simulink model "Stirred_tank_heater_FLC_Xilinx"  (R2017b)
settings: Solver=VariableStepAuto  StartTime=0.0  StopTime=4  RelTol=1e-3
libraries: xbsIndex_r4 x251
(part 1 of 2)
settings Model: Creator=HP  LastModifiedBy=HP

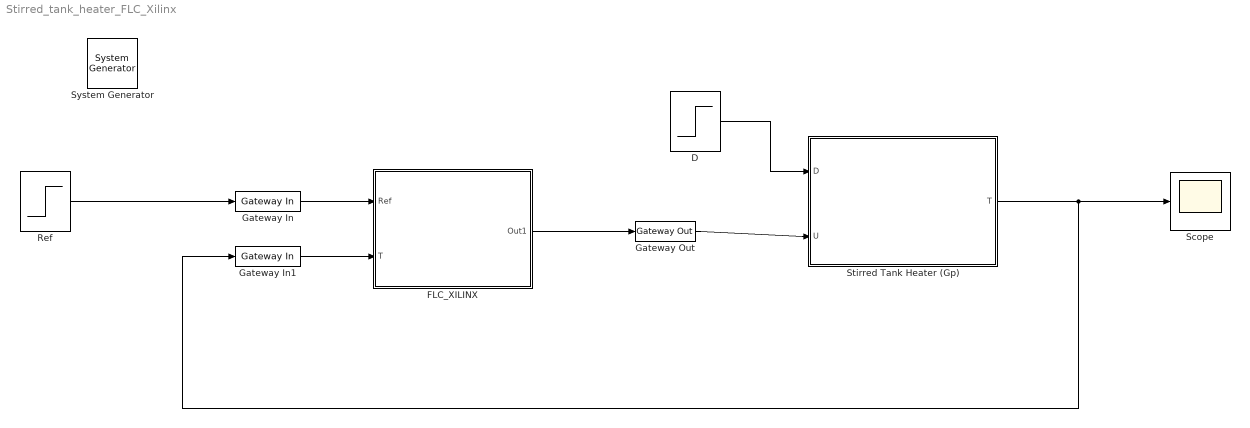
== system Stirred_tank_heater_FLC_Xilinx ==
  " System Generator" : xbsIndex_r4/ System Generator  Tag=genX  xilinxfamily=kintex7  part=xc7k325t  speed=-3  package=fbg676  synthesis_tool=Vivado  clock_wrapper=Clock Enables  directory=./netlist  proj_type=Vivado  Synth_file=Vivado Synthesis Defaults  Impl_file=Vivado Implementation Defaults  testbench=off  simulink_period=1/10e4  sysclk_period=10  dcm_input_clock_period=10  incr_netlist=off  trim_vbits=Everywhere in SubSystem  dbl_ovrd=According to Block Masks  core_generation=According to Block Masks  run_coregen=off  deprecated_control=off  eval_field=0  block_type=sysgen
  D : Step  Time=2  After=0  SampleTime=0.01
  FLC_XILINX : Subsystem
  Gateway In : xbsIndex_r4/Gateway In  gui_display_data_type=Floating-point  arith_type=Floating-point  n_bits=16  bin_pt=14  preci_type=Double  exp_width=8  frac_width=24  rows=1  columns=1  quantization="Round  (unbiased: +/- Inf)"  overflow=Saturate  period=1/10e4  UseAsADC=off  ADCChannel='1'  interface=None  automatic_assignment=on  address_offset=hex2dec('00')  intf_name=''  intf_description=''  default_value=0  timing_constraint=None  locs_specified=off  LOCs={}  io_standard={}  inherit_from_input=off  hdl_port=on  dbl_ovrd=off  block_type=gatewayin
  Gateway In1 : xbsIndex_r4/Gateway In  gui_display_data_type=Floating-point  arith_type=Floating-point  n_bits=16  bin_pt=14  preci_type=Double  exp_width=8  frac_width=24  rows=1  columns=1  quantization="Round  (unbiased: +/- Inf)"  overflow=Saturate  period=1/10e4  UseAsADC=off  ADCChannel='1'  interface=None  automatic_assignment=on  address_offset=hex2dec('00')  intf_name=''  intf_description=''  default_value=0  timing_constraint=None  locs_specified=off  LOCs={}  io_standard={}  inherit_from_input=off  hdl_port=on  dbl_ovrd=off  block_type=gatewayin
  Gateway Out : xbsIndex_r4/Gateway Out  inherit_from_input=off  hdl_port=on  rows=1  columns=1  UseAsDAC=off  DACChannel='1'  interface=None  automatic_assignment=on  address_offset=hex2dec('00')  intf_name=''  intf_description=''  timing_constraint=None  locs_specified=off  LOCs={}  io_standard={}  block_type=gatewayout
  Ref : Step  Time=0  SampleTime=0.01
  Scope : Scope
  Stirred Tank Heater (Gp) : Subsystem
  wires:
  FLC_XILINX/1(Out1) -> Gateway Out/1
  Ref/1 -> Gateway In/1
  Gateway In/1 -> FLC_XILINX/1(Ref)
  Stirred Tank Heater (Gp)/1(T) -> Gateway In1/1, Scope/1
  D/1 -> Stirred Tank Heater (Gp)/1(D)
  Gateway Out/1 -> Stirred Tank Heater (Gp)/2(U)
  Gateway In1/1 -> FLC_XILINX/2(T)

== system Stirred_tank_heater_FLC_Xilinx/FLC_XILINX ==
  Ref : Inport
  T : Inport  Port=2
  AddSub2 : xbsIndex_r4/AddSub  mode=Subtraction  use_carryin=off  use_carryout=off  en=off  latency=1  precision=Full  arith_type=Unsigned  n_bits=16  bin_pt=14  quantization=Truncate  overflow=Wrap  use_behavioral_HDL=off  hw_selection=Fabric  pipelined=off  dbl_ovrd=off  block_type=addsub
  CMult1 : xbsIndex_r4/CMult  const=1/12  gui_display_data_type=Floating-point  const_n_bits=16  const_bin_pt=14  float_type=Double  exp_bits=8  fraction_bits=24  en=off  latency=1  precision=Full  arith_type="Signed  (2's comp)"  n_bits=16  bin_pt=14  quantization=Truncate  overflow=Wrap  use_behavioral_HDL=off  mem_type=Distributed RAM  pipeline=off  dbl_ovrd=off  block_type=cmult
  CMult2 : xbsIndex_r4/CMult  const=36  gui_display_data_type=Floating-point  const_n_bits=16  const_bin_pt=14  float_type=Double  exp_bits=8  fraction_bits=24  en=off  latency=1  precision=Full  arith_type="Signed  (2's comp)"  n_bits=16  bin_pt=14  quantization=Truncate  overflow=Wrap  use_behavioral_HDL=off  mem_type=Distributed RAM  pipeline=off  dbl_ovrd=off  block_type=cmult
  CMult3 : xbsIndex_r4/CMult  const=1  gui_display_data_type=Floating-point  const_n_bits=16  const_bin_pt=14  float_type=Double  exp_bits=8  fraction_bits=24  en=off  latency=1  precision=Full  arith_type="Signed  (2's comp)"  n_bits=16  bin_pt=14  quantization=Truncate  overflow=Wrap  use_behavioral_HDL=off  mem_type=Distributed RAM  pipeline=off  dbl_ovrd=off  block_type=cmult
  Deffuzification : Subsystem
  Input Membership func : Subsystem
  Integrator : Subsystem
  Rules decision logic : Subsystem
  derivative : Subsystem
  Out1 : Outport
  wires:
  Input Membership func/4(PS1) -> Rules decision logic/4(PS1)
  Input Membership func/5(PB1) -> Rules decision logic/5(PB1)
  Input Membership func/6(NB2) -> Rules decision logic/6(NB2)
  Input Membership func/8(ZE2) -> Rules decision logic/8(ZE2)
  Rules decision logic/2(NS3) -> Deffuzification/2(NS3)
  Input Membership func/7(NS2) -> Rules decision logic/7(NS2)
  Input Membership func/1(NB1) -> Rules decision logic/1(NB1)
  Rules decision logic/4(PS3) -> Deffuzification/4(PS3)
  Input Membership func/3(ZE1) -> Rules decision logic/3(ZE1)
  Rules decision logic/3(ZE3) -> Deffuzification/3(ZE3)
  Rules decision logic/5(PB3) -> Deffuzification/5(PB3)
  Input Membership func/2(NS1) -> Rules decision logic/2(NS1)
  Input Membership func/10(PB2) -> Rules decision logic/10(PB2)
  Rules decision logic/1(NB3) -> Deffuzification/1(NB3)
  Input Membership func/9(PS2) -> Rules decision logic/9(PS2)
  Deffuzification/1(du) -> CMult2/1
  Integrator/1(u) -> Out1/1
  CMult2/1 -> Integrator/1(du)
  Ref/1 -> AddSub2/1
  AddSub2/1 -> CMult3/1, derivative/1(du)
  T/1 -> AddSub2/2
  CMult1/1 -> Input Membership func/2(de)
  derivative/1(u) -> CMult1/1
  CMult3/1 -> Input Membership func/1(e)

== system Stirred_tank_heater_FLC_Xilinx/Stirred Tank Heater (Gp) ==
  D : Inport
  U : Inport  Port=2
  Add : Sum
  Transfer Fcn : TransferFcn  Numerator=[3]  Denominator=[1 5]
  Transfer Fcn1 : TransferFcn  Numerator=[2]  Denominator=[1 5]
  T : Outport
  wires:
  U/1 -> Transfer Fcn/1
  Add/1 -> T/1
  Transfer Fcn/1 -> Add/2
  Transfer Fcn1/1 -> Add/1
  D/1 -> Transfer Fcn1/1

== system Stirred_tank_heater_FLC_Xilinx/FLC_XILINX/Deffuzification ==
  NB3 : Inport
  NS3 : Inport  Port=2
  ZE3 : Inport  Port=3
  PS3 : Inport  Port=4
  PB3 : Inport  Port=5
  Constant : xbsIndex_r4/Constant  const=0  gui_display_data_type=Floating-point  arith_type=Floating-point  n_bits=16  bin_pt=14  preci_type=Double  exp_width=8  frac_width=24  explicit_period=off  period=1  equ=P=C  opselect=C  inp2=PCIN>>17  opr=+  inp1=P  carry=CIN  dbl_ovrd=off  block_type=constant
  Constant1 : xbsIndex_r4/Constant  const=0  gui_display_data_type=Floating-point  arith_type=Floating-point  n_bits=16  bin_pt=14  preci_type=Double  exp_width=8  frac_width=24  explicit_period=off  period=1  equ=P=C  opselect=C  inp2=PCIN>>17  opr=+  inp1=P  carry=CIN  dbl_ovrd=off  block_type=constant
  Denum : Subsystem
  Denum1 : Subsystem
  Divide : xbsIndex_r4/Divide  flow_control=NonBlocking  axi_optimize_goal=Resources  algorithm_type=Radix2  infoedit1=Specify output fraction-width for Fixed-point division.  fractional_width=16  infoedit2=Specify latency for Floating-point division.  latency=1  rate=1  has_a_tlast=off  has_a_tuser=off  has_b_tlast=off  has_b_tuser=off  en=off  has_result_tready=off  result_tlast_behv=Pass_A_TLAST  has_underflow=off  has_overflow=off  has_invalid_op=off  has_divide_by_zero=off  fpo_op_type=mergeddivide  block_type=divide
      settings: infoedit=Blocking: Wait for data on all inputs, allow back-pressure.<br>NonBlocking: operate every cycle in which all inputs are valid, no back-pressure.
  Mux : xbsIndex_r4/Mux  inputs=2  en=off  latency=1  precision=Full  arith_type=Unsigned  n_bits=16  bin_pt=14  quantization=Truncate  overflow=Wrap  dbl_ovrd=off  block_type=mux
  Relational : xbsIndex_r4/Relational  mode=a!=b  op_type=Bool  en=off  latency=1  dbl_ovrd=off  block_type=relational
  du : Outport
  wires:
  NB3/1 -> Denum/1(NB3), Denum1/1(NB3)
  NS3/1 -> Denum/2(NS3), Denum1/2(NS3)
  PB3/1 -> Denum/5(PB3), Denum1/4(PB3)
  Constant/1 -> Relational/2
  Relational/1 -> Mux/1
  Constant1/1 -> Mux/2
  ZE3/1 -> Denum/3(ZE3)
  PS3/1 -> Denum/4(PS3), Denum1/3(PS3)
  Denum/1(A6) -> Relational/1, Divide/2
  Denum1/1(N) -> Divide/1
  Divide/1 -> Mux/3
  Mux/1 -> du/1

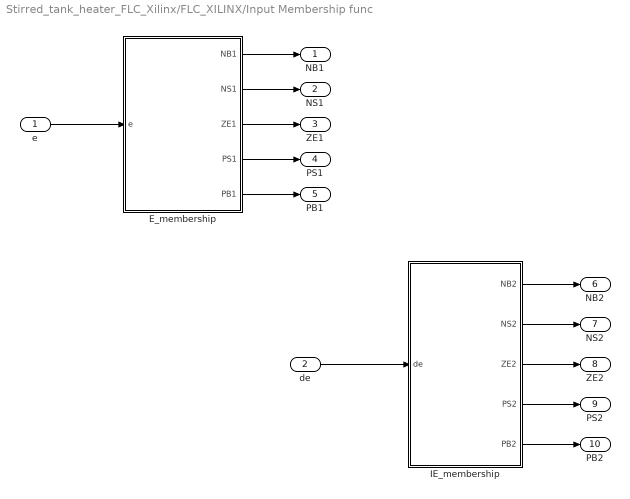
== system Stirred_tank_heater_FLC_Xilinx/FLC_XILINX/Input Membership func ==
  e : Inport
  de : Inport  Port=2
  E_membership : Subsystem
  IE_membership : Subsystem
  NB1 : Outport
  NS1 : Outport  Port=2
  ZE1 : Outport  Port=3
  PS1 : Outport  Port=4
  PB1 : Outport  Port=5
  NB2 : Outport  Port=6
  NS2 : Outport  Port=7
  ZE2 : Outport  Port=8
  PS2 : Outport  Port=9
  PB2 : Outport  Port=10
  wires:
  E_membership/4(PS1) -> PS1/1
  E_membership/2(NS1) -> NS1/1
  E_membership/1(NB1) -> NB1/1
  E_membership/3(ZE1) -> ZE1/1
  e/1 -> E_membership/1(e)
  IE_membership/5(PB2) -> PB2/1
  IE_membership/3(ZE2) -> ZE2/1
  IE_membership/4(PS2) -> PS2/1
  IE_membership/2(NS2) -> NS2/1
  IE_membership/1(NB2) -> NB2/1
  de/1 -> IE_membership/1(de)
  E_membership/5(PB1) -> PB1/1

== system Stirred_tank_heater_FLC_Xilinx/FLC_XILINX/Integrator ==
  du : Inport
  AddSub : xbsIndex_r4/AddSub  mode=Addition  use_carryin=off  use_carryout=off  en=off  latency=0  precision=Full  arith_type=Unsigned  n_bits=16  bin_pt=14  quantization=Truncate  overflow=Wrap  use_behavioral_HDL=off  hw_selection=Fabric  pipelined=off  dbl_ovrd=off  block_type=addsub
  AddSub1 : xbsIndex_r4/AddSub  mode=Addition  use_carryin=off  use_carryout=off  en=off  latency=0  precision=Full  arith_type=Unsigned  n_bits=16  bin_pt=14  quantization=Truncate  overflow=Wrap  use_behavioral_HDL=off  hw_selection=Fabric  pipelined=off  dbl_ovrd=off  block_type=addsub
  CMult : xbsIndex_r4/CMult  const=1/(2*10e4)  gui_display_data_type=Floating-point  const_n_bits=32  const_bin_pt=28  float_type=Double  exp_bits=8  fraction_bits=24  en=off  latency=1  precision=Full  arith_type="Signed  (2's comp)"  n_bits=16  bin_pt=14  quantization=Truncate  overflow=Wrap  use_behavioral_HDL=off  mem_type=Distributed RAM  pipeline=off  dbl_ovrd=off  block_type=cmult
  Delay : xbsIndex_r4/Delay  rst=off  infoeditControl=Selection of Reset will increase slice count due to use of real FFs and instead of SRLs  en=off  latency=1  reg_retiming=off  dbl_ovrd=off  block_type=delay
  Delay1 : xbsIndex_r4/Delay  rst=off  infoeditControl=Selection of Reset will increase slice count due to use of real FFs and instead of SRLs  en=off  latency=1  reg_retiming=off  dbl_ovrd=off  block_type=delay
  u : Outport
  wires:
  CMult/1 -> AddSub1/1
  AddSub1/1 -> u/1, Delay1/1
  AddSub/1 -> CMult/1
  du/1 -> AddSub/1, Delay/1
  Delay/1 -> AddSub/2
  Delay1/1 -> AddSub1/2

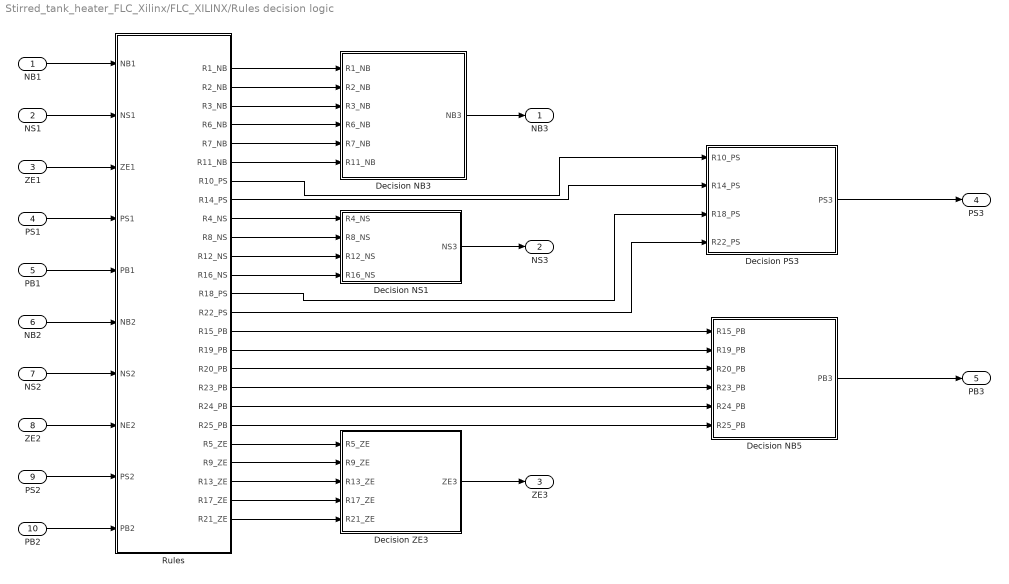
== system Stirred_tank_heater_FLC_Xilinx/FLC_XILINX/Rules decision logic ==
  NB1 : Inport
  NS1 : Inport  Port=2
  ZE1 : Inport  Port=3
  PS1 : Inport  Port=4
  PB1 : Inport  Port=5
  NB2 : Inport  Port=6
  NS2 : Inport  Port=7
  ZE2 : Inport  Port=8
  PS2 : Inport  Port=9
  PB2 : Inport  Port=10
  Decision NB3 : Subsystem
  Decision NB5 : Subsystem
  Decision NS1 : Subsystem
  Decision PS3 : Subsystem
  Decision ZE3 : Subsystem
  Rules : Subsystem
  NB3 : Outport
  NS3 : Outport  Port=2
  ZE3 : Outport  Port=3
  PS3 : Outport  Port=4
  PB3 : Outport  Port=5
  wires:
  NB1/1 -> Rules/1(NB1)
  NB2/1 -> Rules/6(NB2)
  NS2/1 -> Rules/7(NS2)
  ZE2/1 -> Rules/8(NE2)
  PS2/1 -> Rules/9(PS2)
  PB2/1 -> Rules/10(PB2)
  NS1/1 -> Rules/2(NS1)
  ZE1/1 -> Rules/3(ZE1)
  PS1/1 -> Rules/4(PS1)
  PB1/1 -> Rules/5(PB1)
  Decision NB3/1(NB3) -> NB3/1
  Decision NS1/1(NS3) -> NS3/1
  Decision ZE3/1(ZE3) -> ZE3/1
  Decision PS3/1(PS3) -> PS3/1
  Decision NB5/1(PB3) -> PB3/1
  Rules/1(R1_NB) -> Decision NB3/1(R1_NB)
  Rules/2(R2_NB) -> Decision NB3/2(R2_NB)
  Rules/3(R3_NB) -> Decision NB3/3(R3_NB)
  Rules/4(R6_NB) -> Decision NB3/4(R6_NB)
  Rules/5(R7_NB) -> Decision NB3/5(R7_NB)
  Rules/6(R11_NB) -> Decision NB3/6(R11_NB)
  Rules/25(R21_ZE) -> Decision ZE3/5(R21_ZE)
  Rules/24(R17_ZE) -> Decision ZE3/4(R17_ZE)
  Rules/23(R13_ZE) -> Decision ZE3/3(R13_ZE)
  Rules/22(R9_ZE) -> Decision ZE3/2(R9_ZE)
  Rules/21(R5_ZE) -> Decision ZE3/1(R5_ZE)
  Rules/12(R16_NS) -> Decision NS1/4(R16_NS)
  Rules/11(R12_NS) -> Decision NS1/3(R12_NS)
  Rules/10(R8_NS) -> Decision NS1/2(R8_NS)
  Rules/9(R4_NS) -> Decision NS1/1(R4_NS)
  Rules/20(R25_PB) -> Decision NB5/6(R25_PB)
  Rules/19(R24_PB) -> Decision NB5/5(R24_PB)
  Rules/18(R23_PB) -> Decision NB5/4(R23_PB)
  Rules/17(R20_PB) -> Decision NB5/3(R20_PB)
  Rules/16(R19_PB) -> Decision NB5/2(R19_PB)
  Rules/15(R15_PB) -> Decision NB5/1(R15_PB)
  Rules/8(R14_PS) -> Decision PS3/2(R14_PS)
  Rules/7(R10_PS) -> Decision PS3/1(R10_PS)
  Rules/14(R22_PS) -> Decision PS3/4(R22_PS)
  Rules/13(R18_PS) -> Decision PS3/3(R18_PS)

== system Stirred_tank_heater_FLC_Xilinx/FLC_XILINX/derivative ==
  du : Inport
  AddSub2 : xbsIndex_r4/AddSub  mode=Subtraction  use_carryin=off  use_carryout=off  en=off  latency=1  precision=Full  arith_type=Unsigned  n_bits=16  bin_pt=14  quantization=Truncate  overflow=Wrap  use_behavioral_HDL=off  hw_selection=Fabric  pipelined=off  dbl_ovrd=off  block_type=addsub
  CMult2 : xbsIndex_r4/CMult  const=10e4  gui_display_data_type=Floating-point  const_n_bits=16  const_bin_pt=14  float_type=Double  exp_bits=8  fraction_bits=24  en=off  latency=1  precision=Full  arith_type="Signed  (2's comp)"  n_bits=16  bin_pt=14  quantization=Truncate  overflow=Wrap  use_behavioral_HDL=off  mem_type=Distributed RAM  pipeline=off  dbl_ovrd=off  block_type=cmult
  Delay1 : xbsIndex_r4/Delay  rst=off  infoeditControl=Selection of Reset will increase slice count due to use of real FFs and instead of SRLs  en=off  latency=1  reg_retiming=off  dbl_ovrd=off  block_type=delay
  u : Outport
  wires:
  AddSub2/1 -> CMult2/1
  du/1 -> Delay1/1, AddSub2/1
  Delay1/1 -> AddSub2/2
  CMult2/1 -> u/1

== system Stirred_tank_heater_FLC_Xilinx/FLC_XILINX/Deffuzification/Denum ==
  NB3 : Inport
  NS3 : Inport  Port=2
  ZE3 : Inport  Port=3
  PS3 : Inport  Port=4
  PB3 : Inport  Port=5
  AddSub{,1..3} (4 alike) : xbsIndex_r4/AddSub  mode=Addition  use_carryin=off  use_carryout=off  en=off  latency=1  precision=Full  arith_type=Unsigned  n_bits=16  bin_pt=14  quantization=Truncate  overflow=Wrap  use_behavioral_HDL=off  hw_selection=Fabric  pipelined=off  dbl_ovrd=off  block_type=addsub
  A6 : Outport
  wires:
  AddSub1/1 -> AddSub2/1
  AddSub/1 -> AddSub1/1
  AddSub2/1 -> AddSub3/1
  NB3/1 -> AddSub/1
  AddSub3/1 -> A6/1
  PB3/1 -> AddSub3/2
  PS3/1 -> AddSub2/2
  ZE3/1 -> AddSub1/2
  NS3/1 -> AddSub/2

== system Stirred_tank_heater_FLC_Xilinx/FLC_XILINX/Deffuzification/Denum1 ==
  NB3 : Inport
  NS3 : Inport  Port=2
  PS3 : Inport  Port=3
  PB3 : Inport  Port=4
  AddSub : xbsIndex_r4/AddSub  mode=Addition  use_carryin=off  use_carryout=off  en=off  latency=1  precision=Full  arith_type=Unsigned  n_bits=16  bin_pt=14  quantization=Truncate  overflow=Wrap  use_behavioral_HDL=off  hw_selection=Fabric  pipelined=off  dbl_ovrd=off  block_type=addsub
  AddSub1 : xbsIndex_r4/AddSub  mode=Subtraction  use_carryin=off  use_carryout=off  en=off  latency=1  precision=Full  arith_type=Unsigned  n_bits=16  bin_pt=14  quantization=Truncate  overflow=Wrap  use_behavioral_HDL=off  hw_selection=Fabric  pipelined=off  dbl_ovrd=off  block_type=addsub
  AddSub2 : xbsIndex_r4/AddSub  mode=Subtraction  use_carryin=off  use_carryout=off  en=off  latency=1  precision=Full  arith_type=Unsigned  n_bits=16  bin_pt=14  quantization=Truncate  overflow=Wrap  use_behavioral_HDL=off  hw_selection=Fabric  pipelined=off  dbl_ovrd=off  block_type=addsub
  CMult : xbsIndex_r4/CMult  const=10  gui_display_data_type=Floating-point  const_n_bits=16  const_bin_pt=14  float_type=Double  exp_bits=8  fraction_bits=24  en=off  latency=1  precision=Full  arith_type="Signed  (2's comp)"  n_bits=16  bin_pt=14  quantization=Truncate  overflow=Wrap  use_behavioral_HDL=off  mem_type=Distributed RAM  pipeline=off  dbl_ovrd=off  block_type=cmult
  CMult1 : xbsIndex_r4/CMult  const=2  gui_display_data_type=Floating-point  const_n_bits=16  const_bin_pt=14  float_type=Double  exp_bits=8  fraction_bits=24  en=off  latency=1  precision=Full  arith_type="Signed  (2's comp)"  n_bits=16  bin_pt=14  quantization=Truncate  overflow=Wrap  use_behavioral_HDL=off  mem_type=Distributed RAM  pipeline=off  dbl_ovrd=off  block_type=cmult
  CMult2 : xbsIndex_r4/CMult  const=2  gui_display_data_type=Floating-point  const_n_bits=16  const_bin_pt=14  float_type=Double  exp_bits=8  fraction_bits=24  en=off  latency=1  precision=Full  arith_type="Signed  (2's comp)"  n_bits=16  bin_pt=14  quantization=Truncate  overflow=Wrap  use_behavioral_HDL=off  mem_type=Distributed RAM  pipeline=off  dbl_ovrd=off  block_type=cmult
  N : Outport
  wires:
  AddSub1/1 -> AddSub2/1
  AddSub/1 -> AddSub1/1
  AddSub2/1 -> CMult/1
  CMult/1 -> N/1
  CMult1/1 -> AddSub2/2
  PB3/1 -> CMult2/1
  CMult2/1 -> AddSub/1
  PS3/1 -> AddSub/2
  NS3/1 -> AddSub1/2
  NB3/1 -> CMult1/1

== system Stirred_tank_heater_FLC_Xilinx/FLC_XILINX/Input Membership func/E_membership ==
  e : Inport
  NB : Subsystem
  NS : Subsystem
  PB : Subsystem
  PS : Subsystem
  ZE : Subsystem
  NB1 : Outport
  NS1 : Outport  Port=2
  ZE1 : Outport  Port=3
  PS1 : Outport  Port=4
  PB1 : Outport  Port=5
  wires:
  ZE/1(ZE) -> ZE1/1
  PB/1(PB) -> PB1/1
  PS/1(PS) -> PS1/1
  e/1 -> PB/1(e), PS/1(e), ZE/1(e), NS/1(e), NB/1(e)
  NB/1(NB) -> NB1/1
  NS/1(NS) -> NS1/1

== system Stirred_tank_heater_FLC_Xilinx/FLC_XILINX/Input Membership func/IE_membership ==
  de : Inport
  NB : Subsystem
  NS : Subsystem
  PB : Subsystem
  PS : Subsystem
  ZE : Subsystem
  NB2 : Outport
  NS2 : Outport  Port=2
  ZE2 : Outport  Port=3
  PS2 : Outport  Port=4
  PB2 : Outport  Port=5
  wires:
  ZE/1(ZE) -> ZE2/1
  PB/1(PB) -> PB2/1
  PS/1(PS) -> PS2/1
  de/1 -> NB/1(de), NS/1(de), ZE/1(de), PS/1(de), PB/1(de)
  NB/1(NB) -> NB2/1
  NS/1(NS) -> NS2/1

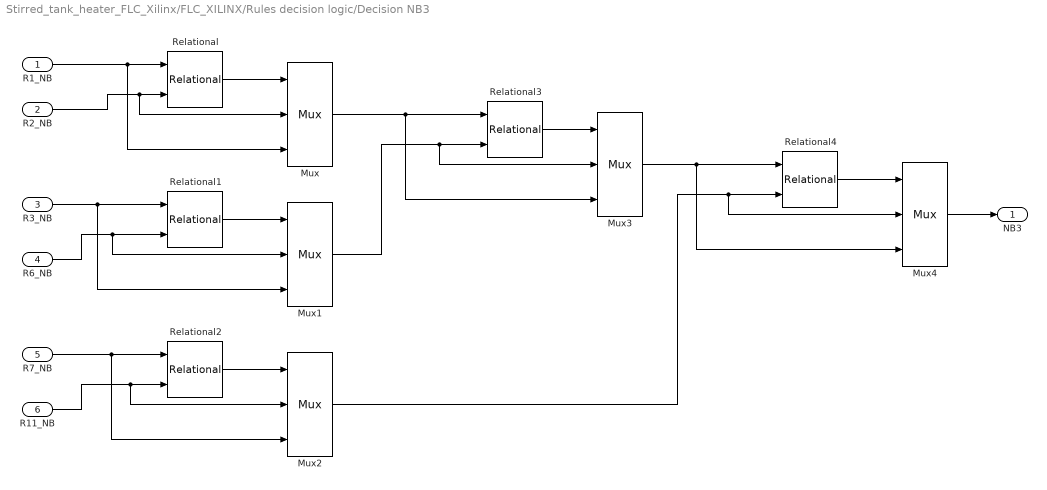
== system Stirred_tank_heater_FLC_Xilinx/FLC_XILINX/Rules decision logic/Decision NB3 ==
  R1_NB : Inport
  R2_NB : Inport  Port=2
  R3_NB : Inport  Port=3
  R6_NB : Inport  Port=4
  R7_NB : Inport  Port=5
  R11_NB : Inport  Port=6
  Mux{,1..4} (5 alike) : xbsIndex_r4/Mux  inputs=2  en=off  latency=1  precision=Full  arith_type=Unsigned  n_bits=16  bin_pt=14  quantization=Truncate  overflow=Wrap  dbl_ovrd=off  block_type=mux
  Relational{,1..4} (5 alike) : xbsIndex_r4/Relational  mode=a>b  op_type=Bool  en=off  latency=1  dbl_ovrd=off  block_type=relational
  NB3 : Outport
  wires:
  R1_NB/1 -> Relational/1, Mux/3
  R2_NB/1 -> Relational/2, Mux/2
  Relational/1 -> Mux/1
  Relational1/1 -> Mux1/1
  R6_NB/1 -> Mux1/2, Relational1/2
  R3_NB/1 -> Mux1/3, Relational1/1
  Relational2/1 -> Mux2/1
  R11_NB/1 -> Mux2/2, Relational2/2
  R7_NB/1 -> Mux2/3, Relational2/1
  Relational3/1 -> Mux3/1
  Mux/1 -> Relational3/1, Mux3/3
  Mux1/1 -> Relational3/2, Mux3/2
  Relational4/1 -> Mux4/1
  Mux3/1 -> Mux4/3, Relational4/1
  Mux2/1 -> Mux4/2, Relational4/2
  Mux4/1 -> NB3/1

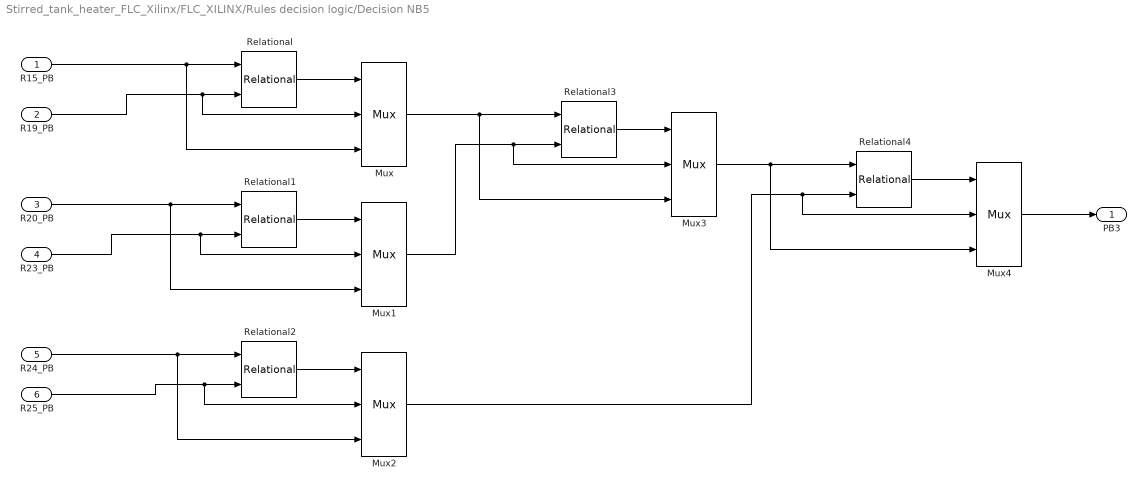
== system Stirred_tank_heater_FLC_Xilinx/FLC_XILINX/Rules decision logic/Decision NB5 ==
  R15_PB : Inport
  R19_PB : Inport  Port=2
  R20_PB : Inport  Port=3
  R23_PB : Inport  Port=4
  R24_PB : Inport  Port=5
  R25_PB : Inport  Port=6
  Mux{,1..4} (5 alike) : xbsIndex_r4/Mux  inputs=2  en=off  latency=1  precision=Full  arith_type=Unsigned  n_bits=16  bin_pt=14  quantization=Truncate  overflow=Wrap  dbl_ovrd=off  block_type=mux
  Relational{,1..4} (5 alike) : xbsIndex_r4/Relational  mode=a>b  op_type=Bool  en=off  latency=1  dbl_ovrd=off  block_type=relational
  PB3 : Outport
  wires:
  Mux/1 -> Relational3/1, Mux3/3
  R15_PB/1 -> Relational/1, Mux/3
  Relational/1 -> Mux/1
  R19_PB/1 -> Relational/2, Mux/2
  R25_PB/1 -> Mux2/2, Relational2/2
  Relational4/1 -> Mux4/1
  Mux3/1 -> Mux4/3, Relational4/1
  Relational2/1 -> Mux2/1
  Relational1/1 -> Mux1/1
  R20_PB/1 -> Mux1/3, Relational1/1
  Mux2/1 -> Mux4/2, Relational4/2
  Mux1/1 -> Relational3/2, Mux3/2
  Relational3/1 -> Mux3/1
  R24_PB/1 -> Mux2/3, Relational2/1
  Mux4/1 -> PB3/1
  R23_PB/1 -> Mux1/2, Relational1/2

== system Stirred_tank_heater_FLC_Xilinx/FLC_XILINX/Rules decision logic/Decision NS1 ==
  R4_NS : Inport
  R8_NS : Inport  Port=2
  R12_NS : Inport  Port=3
  R16_NS : Inport  Port=4
  Mux : xbsIndex_r4/Mux  inputs=2  en=off  latency=1  precision=Full  arith_type=Unsigned  n_bits=16  bin_pt=14  quantization=Truncate  overflow=Wrap  dbl_ovrd=off  block_type=mux
  Mux1 : xbsIndex_r4/Mux  inputs=2  en=off  latency=1  precision=Full  arith_type=Unsigned  n_bits=16  bin_pt=14  quantization=Truncate  overflow=Wrap  dbl_ovrd=off  block_type=mux
  Mux3 : xbsIndex_r4/Mux  inputs=2  en=off  latency=1  precision=Full  arith_type=Unsigned  n_bits=16  bin_pt=14  quantization=Truncate  overflow=Wrap  dbl_ovrd=off  block_type=mux
  Relational : xbsIndex_r4/Relational  mode=a>b  op_type=Bool  en=off  latency=1  dbl_ovrd=off  block_type=relational
  Relational1 : xbsIndex_r4/Relational  mode=a>b  op_type=Bool  en=off  latency=1  dbl_ovrd=off  block_type=relational
  Relational3 : xbsIndex_r4/Relational  mode=a>b  op_type=Bool  en=off  latency=1  dbl_ovrd=off  block_type=relational
  NS3 : Outport
  wires:
  Relational3/1 -> Mux3/1
  Relational/1 -> Mux/1
  Mux/1 -> Relational3/1, Mux3/3
  R8_NS/1 -> Relational/2, Mux/2
  R4_NS/1 -> Relational/1, Mux/3
  Mux3/1 -> NS3/1
  R12_NS/1 -> Mux1/3, Relational1/1
  R16_NS/1 -> Relational1/2, Mux1/2
  Relational1/1 -> Mux1/1
  Mux1/1 -> Mux3/2, Relational3/2

== system Stirred_tank_heater_FLC_Xilinx/FLC_XILINX/Rules decision logic/Decision PS3 ==
  R10_PS : Inport
  R14_PS : Inport  Port=2
  R18_PS : Inport  Port=3
  R22_PS : Inport  Port=4
  Mux : xbsIndex_r4/Mux  inputs=2  en=off  latency=1  precision=Full  arith_type=Unsigned  n_bits=16  bin_pt=14  quantization=Truncate  overflow=Wrap  dbl_ovrd=off  block_type=mux
  Mux1 : xbsIndex_r4/Mux  inputs=2  en=off  latency=1  precision=Full  arith_type=Unsigned  n_bits=16  bin_pt=14  quantization=Truncate  overflow=Wrap  dbl_ovrd=off  block_type=mux
  Mux3 : xbsIndex_r4/Mux  inputs=2  en=off  latency=1  precision=Full  arith_type=Unsigned  n_bits=16  bin_pt=14  quantization=Truncate  overflow=Wrap  dbl_ovrd=off  block_type=mux
  Relational : xbsIndex_r4/Relational  mode=a>b  op_type=Bool  en=off  latency=1  dbl_ovrd=off  block_type=relational
  Relational1 : xbsIndex_r4/Relational  mode=a>b  op_type=Bool  en=off  latency=1  dbl_ovrd=off  block_type=relational
  Relational3 : xbsIndex_r4/Relational  mode=a>b  op_type=Bool  en=off  latency=1  dbl_ovrd=off  block_type=relational
  PS3 : Outport
  wires:
  Relational3/1 -> Mux3/1
  Relational/1 -> Mux/1
  Relational1/1 -> Mux1/1
  Mux/1 -> Relational3/1, Mux3/3
  R22_PS/1 -> Relational1/2, Mux1/2
  Mux1/1 -> Relational3/2, Mux3/2
  R14_PS/1 -> Relational/2, Mux/2
  R10_PS/1 -> Relational/1, Mux/3
  Mux3/1 -> PS3/1
  R18_PS/1 -> Relational1/1, Mux1/3

== system Stirred_tank_heater_FLC_Xilinx/FLC_XILINX/Rules decision logic/Decision ZE3 ==
  R5_ZE : Inport
  R9_ZE : Inport  Port=2
  R13_ZE : Inport  Port=3
  R17_ZE : Inport  Port=4
  R21_ZE : Inport  Port=5
  Mux{,1,3..4} (4 alike) : xbsIndex_r4/Mux  inputs=2  en=off  latency=1  precision=Full  arith_type=Unsigned  n_bits=16  bin_pt=14  quantization=Truncate  overflow=Wrap  dbl_ovrd=off  block_type=mux
  Relational{,1,3..4} (4 alike) : xbsIndex_r4/Relational  mode=a>b  op_type=Bool  en=off  latency=1  dbl_ovrd=off  block_type=relational
  ZE3 : Outport
  wires:
  R17_ZE/1 -> Mux1/2, Relational1/2
  Mux/1 -> Relational3/1, Mux3/3
  R5_ZE/1 -> Relational/1, Mux/3
  R9_ZE/1 -> Relational/2, Mux/2
  Relational4/1 -> Mux4/1
  Mux3/1 -> Mux4/3, Relational4/1
  R13_ZE/1 -> Mux1/3, Relational1/1
  Relational1/1 -> Mux1/1
  Mux4/1 -> ZE3/1
  Relational/1 -> Mux/1
  R21_ZE/1 -> Mux4/2, Relational4/2
  Mux1/1 -> Relational3/2, Mux3/2
  Relational3/1 -> Mux3/1

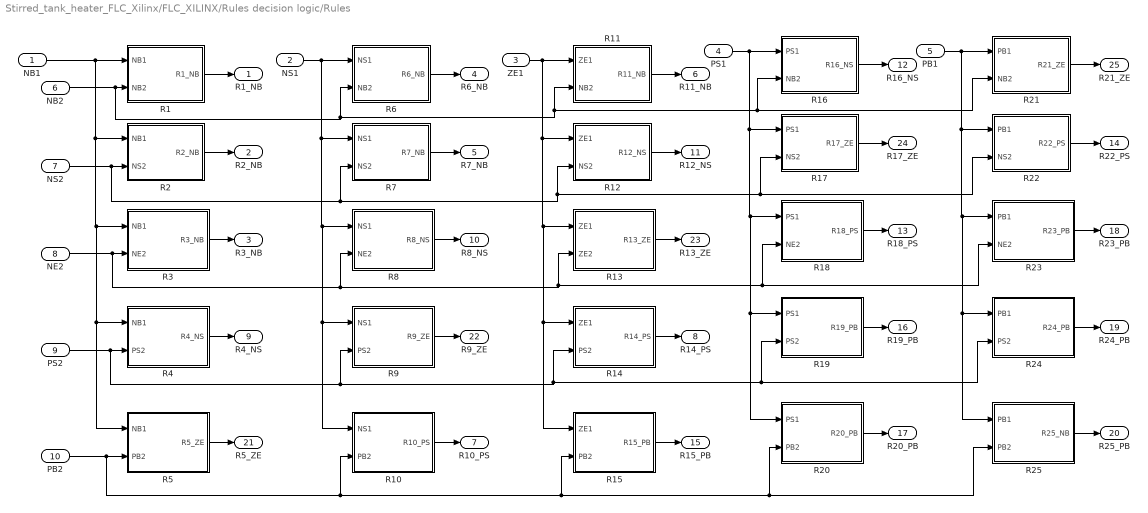
== system Stirred_tank_heater_FLC_Xilinx/FLC_XILINX/Rules decision logic/Rules ==
  NB1 : Inport
  NS1 : Inport  Port=2
  ZE1 : Inport  Port=3
  PS1 : Inport  Port=4
  PB1 : Inport  Port=5
  NB2 : Inport  Port=6
  NS2 : Inport  Port=7
  NE2 : Inport  Port=8
  PS2 : Inport  Port=9
  PB2 : Inport  Port=10
  R1 : Subsystem
  R10 : Subsystem
  R11 : Subsystem
  R12 : Subsystem
  R13 : Subsystem
  R14 : Subsystem
  R15 : Subsystem
  R16 : Subsystem
  R17 : Subsystem
  R18 : Subsystem
  R19 : Subsystem
  R2 : Subsystem
  R20 : Subsystem
  R21 : Subsystem
  R22 : Subsystem
  R23 : Subsystem
  R24 : Subsystem
  R25 : Subsystem
  R3 : Subsystem
  R4 : Subsystem
  R5 : Subsystem
  R6 : Subsystem
  R7 : Subsystem
  R8 : Subsystem
  R9 : Subsystem
  R1_NB : Outport
  R2_NB : Outport  Port=2
  R3_NB : Outport  Port=3
  R6_NB : Outport  Port=4
  R7_NB : Outport  Port=5
  R11_NB : Outport  Port=6
  R10_PS : Outport  Port=7
  R14_PS : Outport  Port=8
  R4_NS : Outport  Port=9
  R8_NS : Outport  Port=10
  R12_NS : Outport  Port=11
  R16_NS : Outport  Port=12
  R18_PS : Outport  Port=13
  R22_PS : Outport  Port=14
  R15_PB : Outport  Port=15
  R19_PB : Outport  Port=16
  R20_PB : Outport  Port=17
  R23_PB : Outport  Port=18
  R24_PB : Outport  Port=19
  R25_PB : Outport  Port=20
  R5_ZE : Outport  Port=21
  R9_ZE : Outport  Port=22
  R13_ZE : Outport  Port=23
  R17_ZE : Outport  Port=24
  R21_ZE : Outport  Port=25
  wires:
  R1/1(R1_NB) -> R1_NB/1
  NB1/1 -> R3/1(NB1), R4/1(NB1), R5/1(NB1), R2/1(NB1), R1/1(NB1)
  R2/1(R2_NB) -> R2_NB/1
  R3/1(R3_NB) -> R3_NB/1
  R4/1(R4_NS) -> R4_NS/1
  R5/1(R5_ZE) -> R5_ZE/1
  R9/1(R9_ZE) -> R9_ZE/1
  R7/1(R7_NB) -> R7_NB/1
  R8/1(R8_NS) -> R8_NS/1
  R10/1(R10_PS) -> R10_PS/1
  NS1/1 -> R8/1(NS1), R9/1(NS1), R10/1(NS1), R7/1(NS1), R6/1(NS1)
  R6/1(R6_NB) -> R6_NB/1
  R14/1(R14_PS) -> R14_PS/1
  R12/1(R12_NS) -> R12_NS/1
  R13/1(R13_ZE) -> R13_ZE/1
  R15/1(R15_PB) -> R15_PB/1
  R11/1(R11_NB) -> R11_NB/1
  R19/1(R19_PB) -> R19_PB/1
  R17/1(R17_ZE) -> R17_ZE/1
  R18/1(R18_PS) -> R18_PS/1
  ZE1/1 -> R13/1(ZE1), R14/1(ZE1), R15/1(ZE1), R12/1(ZE1), R11/1(ZE1)
  R20/1(R20_PB) -> R20_PB/1
  PS1/1 -> R18/1(PS1), R19/1(PS1), R20/1(PS1), R17/1(PS1), R16/1(PS1)
  R16/1(R16_NS) -> R16_NS/1
  R25/1(R25_NB) -> R25_PB/1
  R21/1(R21_ZE) -> R21_ZE/1
  R24/1(R24_PB) -> R24_PB/1
  R23/1(R23_PB) -> R23_PB/1
  R22/1(R22_PS) -> R22_PS/1
  PB2/1 -> R25/2(PB2), R20/2(PB2), R15/2(PB2), R10/2(PB2), R5/2(PB2)
  NE2/1 -> R23/2(NE2), R18/2(NE2), R13/2(ZE2), R8/2(NE2), R3/2(NE2)
  NS2/1 -> R17/2(NS2), R22/2(NS2), R12/2(NS2), R7/2(NS2), R2/2(NS2)
  NB2/1 -> R21/2(NB2), R16/2(NB2), R11/2(NB2), R6/2(NB2), R1/2(NB2)
  PS2/1 -> R9/2(PS2), R14/2(PS2), R24/2(PS2), R19/2(PS2), R4/2(PS2)
  PB1/1 -> R23/1(PB1), R24/1(PB1), R25/1(PB1), R22/1(PB1), R21/1(PB1)

== system Stirred_tank_heater_FLC_Xilinx/FLC_XILINX/Input Membership func/E_membership/NB ==
  e : Inport
  AddSub : xbsIndex_r4/AddSub  mode=Addition  use_carryin=off  use_carryout=off  en=off  latency=1  precision=Full  arith_type=Unsigned  n_bits=16  bin_pt=14  quantization=Truncate  overflow=Wrap  use_behavioral_HDL=off  hw_selection=Fabric  pipelined=off  dbl_ovrd=off  block_type=addsub
  CMult : xbsIndex_r4/CMult  const=-1/5  gui_display_data_type=Floating-point  const_n_bits=16  const_bin_pt=14  float_type=Double  exp_bits=8  fraction_bits=24  en=off  latency=1  precision=Full  arith_type="Signed  (2's comp)"  n_bits=16  bin_pt=14  quantization=Truncate  overflow=Wrap  use_behavioral_HDL=off  mem_type=Distributed RAM  pipeline=off  dbl_ovrd=off  block_type=cmult
  Constant : xbsIndex_r4/Constant  const=-10  gui_display_data_type=Floating-point  arith_type=Floating-point  n_bits=16  bin_pt=14  preci_type=Double  exp_width=8  frac_width=24  explicit_period=off  period=1  equ=P=C  opselect=C  inp2=PCIN>>17  opr=+  inp1=P  carry=CIN  dbl_ovrd=off  block_type=constant
  Constant1 : xbsIndex_r4/Constant  const=-5  gui_display_data_type=Floating-point  arith_type=Floating-point  n_bits=16  bin_pt=14  preci_type=Double  exp_width=8  frac_width=24  explicit_period=off  period=1  equ=P=C  opselect=C  inp2=PCIN>>17  opr=+  inp1=P  carry=CIN  dbl_ovrd=off  block_type=constant
  Constant2 : xbsIndex_r4/Constant  const=5  gui_display_data_type=Floating-point  arith_type=Floating-point  n_bits=16  bin_pt=14  preci_type=Double  exp_width=8  frac_width=24  explicit_period=off  period=1  equ=P=C  opselect=C  inp2=PCIN>>17  opr=+  inp1=P  carry=CIN  dbl_ovrd=off  block_type=constant
  Constant3 : xbsIndex_r4/Constant  const=0  gui_display_data_type=Floating-point  arith_type=Floating-point  n_bits=16  bin_pt=14  preci_type=Double  exp_width=8  frac_width=24  explicit_period=off  period=1  equ=P=C  opselect=C  inp2=PCIN>>17  opr=+  inp1=P  carry=CIN  dbl_ovrd=off  block_type=constant
  Logical : xbsIndex_r4/Logical  logical_function=OR  inputs=2  en=off  latency=1  precision=Full  arith_type=Unsigned  n_bits=16  bin_pt=0  align_bp=on  dbl_ovrd=off  block_type=logical
  Mux : xbsIndex_r4/Mux  inputs=2  en=off  latency=1  precision=Full  arith_type=Unsigned  n_bits=16  bin_pt=14  quantization=Truncate  overflow=Wrap  dbl_ovrd=off  block_type=mux
  Relational : xbsIndex_r4/Relational  mode=a<b  op_type=Bool  en=off  latency=1  dbl_ovrd=off  block_type=relational
  Relational1 : xbsIndex_r4/Relational  mode=a>b  op_type=Bool  en=off  latency=1  dbl_ovrd=off  block_type=relational
  NB : Outport
  wires:
  CMult/1 -> Mux/2
  e/1 -> AddSub/1, Relational1/1, Relational/1
  Constant1/1 -> Relational1/2
  Mux/1 -> NB/1
  Logical/1 -> Mux/1
  Relational/1 -> Logical/1
  Constant/1 -> Relational/2
  Constant3/1 -> Mux/3
  Relational1/1 -> Logical/2
  Constant2/1 -> AddSub/2
  AddSub/1 -> CMult/1

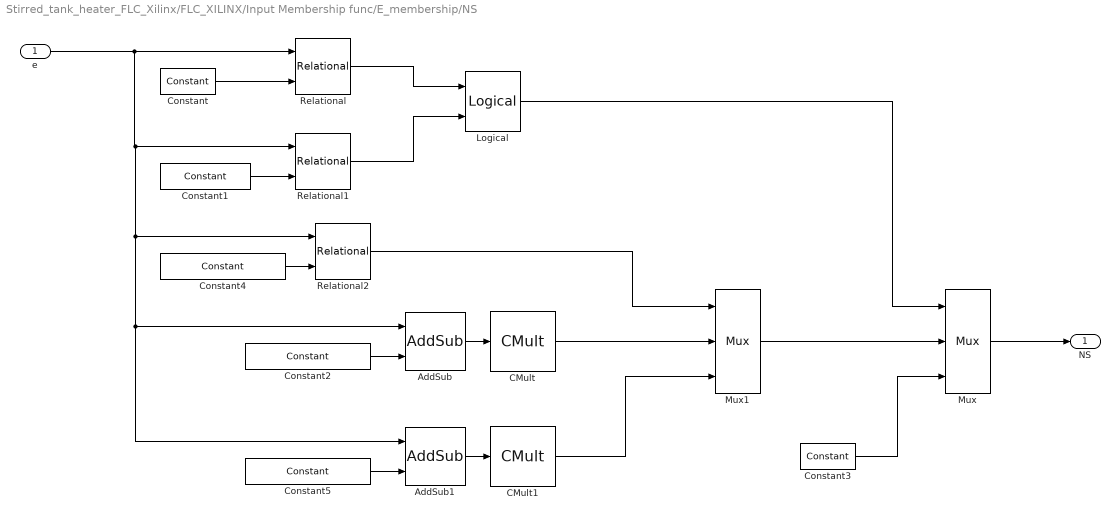
== system Stirred_tank_heater_FLC_Xilinx/FLC_XILINX/Input Membership func/E_membership/NS ==
  e : Inport
  AddSub : xbsIndex_r4/AddSub  mode=Subtraction  use_carryin=off  use_carryout=off  en=off  latency=1  precision=Full  arith_type=Unsigned  n_bits=16  bin_pt=14  quantization=Truncate  overflow=Wrap  use_behavioral_HDL=off  hw_selection=Fabric  pipelined=off  dbl_ovrd=off  block_type=addsub
  AddSub1 : xbsIndex_r4/AddSub  mode=Addition  use_carryin=off  use_carryout=off  en=off  latency=1  precision=Full  arith_type=Unsigned  n_bits=16  bin_pt=14  quantization=Truncate  overflow=Wrap  use_behavioral_HDL=off  hw_selection=Fabric  pipelined=off  dbl_ovrd=off  block_type=addsub
  CMult : xbsIndex_r4/CMult  const=-1/5  gui_display_data_type=Floating-point  const_n_bits=16  const_bin_pt=14  float_type=Double  exp_bits=8  fraction_bits=24  en=off  latency=1  precision=Full  arith_type="Signed  (2's comp)"  n_bits=16  bin_pt=14  quantization=Truncate  overflow=Wrap  use_behavioral_HDL=off  mem_type=Distributed RAM  pipeline=off  dbl_ovrd=off  block_type=cmult
  CMult1 : xbsIndex_r4/CMult  const=1/5  gui_display_data_type=Floating-point  const_n_bits=16  const_bin_pt=14  float_type=Double  exp_bits=8  fraction_bits=24  en=off  latency=1  precision=Full  arith_type="Signed  (2's comp)"  n_bits=16  bin_pt=14  quantization=Truncate  overflow=Wrap  use_behavioral_HDL=off  mem_type=Distributed RAM  pipeline=off  dbl_ovrd=off  block_type=cmult
  Constant : xbsIndex_r4/Constant  const=-10  gui_display_data_type=Floating-point  arith_type=Floating-point  n_bits=16  bin_pt=14  preci_type=Double  exp_width=8  frac_width=24  explicit_period=off  period=1  equ=P=C  opselect=C  inp2=PCIN>>17  opr=+  inp1=P  carry=CIN  dbl_ovrd=off  block_type=constant
  Constant1 : xbsIndex_r4/Constant  const=0  gui_display_data_type=Floating-point  arith_type=Floating-point  n_bits=16  bin_pt=14  preci_type=Double  exp_width=8  frac_width=24  explicit_period=off  period=1  equ=P=C  opselect=C  inp2=PCIN>>17  opr=+  inp1=P  carry=CIN  dbl_ovrd=off  block_type=constant
  Constant2 : xbsIndex_r4/Constant  const=0  gui_display_data_type=Floating-point  arith_type=Floating-point  n_bits=16  bin_pt=14  preci_type=Double  exp_width=8  frac_width=24  explicit_period=off  period=1  equ=P=C  opselect=C  inp2=PCIN>>17  opr=+  inp1=P  carry=CIN  dbl_ovrd=off  block_type=constant
  Constant3 : xbsIndex_r4/Constant  const=0  gui_display_data_type=Floating-point  arith_type=Floating-point  n_bits=16  bin_pt=14  preci_type=Double  exp_width=8  frac_width=24  explicit_period=off  period=1  equ=P=C  opselect=C  inp2=PCIN>>17  opr=+  inp1=P  carry=CIN  dbl_ovrd=off  block_type=constant
  Constant4 : xbsIndex_r4/Constant  const=-5  gui_display_data_type=Floating-point  arith_type=Floating-point  n_bits=16  bin_pt=14  preci_type=Double  exp_width=8  frac_width=24  explicit_period=off  period=1  equ=P=C  opselect=C  inp2=PCIN>>17  opr=+  inp1=P  carry=CIN  dbl_ovrd=off  block_type=constant
  Constant5 : xbsIndex_r4/Constant  const=10  gui_display_data_type=Floating-point  arith_type=Floating-point  n_bits=16  bin_pt=14  preci_type=Double  exp_width=8  frac_width=24  explicit_period=off  period=1  equ=P=C  opselect=C  inp2=PCIN>>17  opr=+  inp1=P  carry=CIN  dbl_ovrd=off  block_type=constant
  Logical : xbsIndex_r4/Logical  logical_function=OR  inputs=2  en=off  latency=1  precision=Full  arith_type=Unsigned  n_bits=16  bin_pt=0  align_bp=on  dbl_ovrd=off  block_type=logical
  Mux : xbsIndex_r4/Mux  inputs=2  en=off  latency=1  precision=Full  arith_type=Unsigned  n_bits=16  bin_pt=14  quantization=Truncate  overflow=Wrap  dbl_ovrd=off  block_type=mux
  Mux1 : xbsIndex_r4/Mux  inputs=2  en=off  latency=1  precision=Full  arith_type=Unsigned  n_bits=16  bin_pt=14  quantization=Truncate  overflow=Wrap  dbl_ovrd=off  block_type=mux
  Relational : xbsIndex_r4/Relational  mode=a<b  op_type=Bool  en=off  latency=1  dbl_ovrd=off  block_type=relational
  Relational1 : xbsIndex_r4/Relational  mode=a>b  op_type=Bool  en=off  latency=1  dbl_ovrd=off  block_type=relational
  Relational2 : xbsIndex_r4/Relational  mode=a<b  op_type=Bool  en=off  latency=1  dbl_ovrd=off  block_type=relational
  NS : Outport
  wires:
  Constant1/1 -> Relational1/2
  Mux/1 -> NS/1
  Logical/1 -> Mux/1
  Relational/1 -> Logical/1
  Constant/1 -> Relational/2
  Constant3/1 -> Mux/3
  Relational1/1 -> Logical/2
  Constant2/1 -> AddSub/2
  AddSub/1 -> CMult/1
  Constant4/1 -> Relational2/2
  Relational2/1 -> Mux1/1
  AddSub1/1 -> CMult1/1
  Constant5/1 -> AddSub1/2
  e/1 -> Relational2/1, AddSub1/1, AddSub/1, Relational1/1, Relational/1
  CMult1/1 -> Mux1/3
  CMult/1 -> Mux1/2
  Mux1/1 -> Mux/2

== system Stirred_tank_heater_FLC_Xilinx/FLC_XILINX/Input Membership func/E_membership/PB ==
  e : Inport
  AddSub : xbsIndex_r4/AddSub  mode=Subtraction  use_carryin=off  use_carryout=off  en=off  latency=1  precision=Full  arith_type=Unsigned  n_bits=16  bin_pt=14  quantization=Truncate  overflow=Wrap  use_behavioral_HDL=off  hw_selection=Fabric  pipelined=off  dbl_ovrd=off  block_type=addsub
  CMult : xbsIndex_r4/CMult  const=1/5  gui_display_data_type=Floating-point  const_n_bits=16  const_bin_pt=14  float_type=Double  exp_bits=8  fraction_bits=24  en=off  latency=1  precision=Full  arith_type="Signed  (2's comp)"  n_bits=16  bin_pt=14  quantization=Truncate  overflow=Wrap  use_behavioral_HDL=off  mem_type=Distributed RAM  pipeline=off  dbl_ovrd=off  block_type=cmult
  Constant : xbsIndex_r4/Constant  const=5  gui_display_data_type=Floating-point  arith_type=Floating-point  n_bits=16  bin_pt=14  preci_type=Double  exp_width=8  frac_width=24  explicit_period=off  period=1  equ=P=C  opselect=C  inp2=PCIN>>17  opr=+  inp1=P  carry=CIN  dbl_ovrd=off  block_type=constant
  Constant1 : xbsIndex_r4/Constant  const=10  gui_display_data_type=Floating-point  arith_type=Floating-point  n_bits=16  bin_pt=14  preci_type=Double  exp_width=8  frac_width=24  explicit_period=off  period=1  equ=P=C  opselect=C  inp2=PCIN>>17  opr=+  inp1=P  carry=CIN  dbl_ovrd=off  block_type=constant
  Constant2 : xbsIndex_r4/Constant  const=10  gui_display_data_type=Floating-point  arith_type=Floating-point  n_bits=16  bin_pt=14  preci_type=Double  exp_width=8  frac_width=24  explicit_period=off  period=1  equ=P=C  opselect=C  inp2=PCIN>>17  opr=+  inp1=P  carry=CIN  dbl_ovrd=off  block_type=constant
  Constant3 : xbsIndex_r4/Constant  const=0  gui_display_data_type=Floating-point  arith_type=Floating-point  n_bits=16  bin_pt=14  preci_type=Double  exp_width=8  frac_width=24  explicit_period=off  period=1  equ=P=C  opselect=C  inp2=PCIN>>17  opr=+  inp1=P  carry=CIN  dbl_ovrd=off  block_type=constant
  Logical : xbsIndex_r4/Logical  logical_function=OR  inputs=2  en=off  latency=1  precision=Full  arith_type=Unsigned  n_bits=16  bin_pt=0  align_bp=on  dbl_ovrd=off  block_type=logical
  Mux : xbsIndex_r4/Mux  inputs=2  en=off  latency=1  precision=Full  arith_type=Unsigned  n_bits=16  bin_pt=14  quantization=Truncate  overflow=Wrap  dbl_ovrd=off  block_type=mux
  Relational : xbsIndex_r4/Relational  mode=a<b  op_type=Bool  en=off  latency=1  dbl_ovrd=off  block_type=relational
  Relational1 : xbsIndex_r4/Relational  mode=a>b  op_type=Bool  en=off  latency=1  dbl_ovrd=off  block_type=relational
  PB : Outport
  wires:
  CMult/1 -> Mux/2
  e/1 -> AddSub/1, Relational1/1, Relational/1
  Constant1/1 -> Relational1/2
  Mux/1 -> PB/1
  Logical/1 -> Mux/1
  Relational/1 -> Logical/1
  Constant/1 -> Relational/2
  Constant3/1 -> Mux/3
  Relational1/1 -> Logical/2
  Constant2/1 -> AddSub/2
  AddSub/1 -> CMult/1

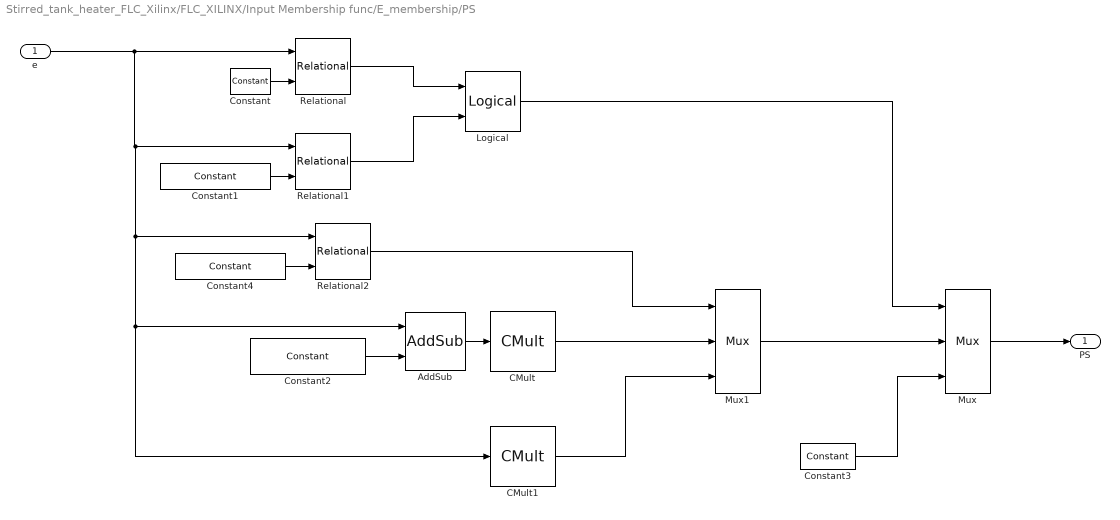
== system Stirred_tank_heater_FLC_Xilinx/FLC_XILINX/Input Membership func/E_membership/PS ==
  e : Inport
  AddSub : xbsIndex_r4/AddSub  mode=Subtraction  use_carryin=off  use_carryout=off  en=off  latency=1  precision=Full  arith_type=Unsigned  n_bits=16  bin_pt=14  quantization=Truncate  overflow=Wrap  use_behavioral_HDL=off  hw_selection=Fabric  pipelined=off  dbl_ovrd=off  block_type=addsub
  CMult : xbsIndex_r4/CMult  const=-1/5  gui_display_data_type=Floating-point  const_n_bits=16  const_bin_pt=14  float_type=Double  exp_bits=8  fraction_bits=24  en=off  latency=1  precision=Full  arith_type="Signed  (2's comp)"  n_bits=16  bin_pt=14  quantization=Truncate  overflow=Wrap  use_behavioral_HDL=off  mem_type=Distributed RAM  pipeline=off  dbl_ovrd=off  block_type=cmult
  CMult1 : xbsIndex_r4/CMult  const=1/5  gui_display_data_type=Floating-point  const_n_bits=16  const_bin_pt=14  float_type=Double  exp_bits=8  fraction_bits=24  en=off  latency=1  precision=Full  arith_type="Signed  (2's comp)"  n_bits=16  bin_pt=14  quantization=Truncate  overflow=Wrap  use_behavioral_HDL=off  mem_type=Distributed RAM  pipeline=off  dbl_ovrd=off  block_type=cmult
  Constant : xbsIndex_r4/Constant  const=0  gui_display_data_type=Floating-point  arith_type=Floating-point  n_bits=16  bin_pt=14  preci_type=Double  exp_width=8  frac_width=24  explicit_period=off  period=1  equ=P=C  opselect=C  inp2=PCIN>>17  opr=+  inp1=P  carry=CIN  dbl_ovrd=off  block_type=constant
  Constant1 : xbsIndex_r4/Constant  const=10  gui_display_data_type=Floating-point  arith_type=Floating-point  n_bits=16  bin_pt=14  preci_type=Double  exp_width=8  frac_width=24  explicit_period=off  period=1  equ=P=C  opselect=C  inp2=PCIN>>17  opr=+  inp1=P  carry=CIN  dbl_ovrd=off  block_type=constant
  Constant2 : xbsIndex_r4/Constant  const=10  gui_display_data_type=Floating-point  arith_type=Floating-point  n_bits=16  bin_pt=14  preci_type=Double  exp_width=8  frac_width=24  explicit_period=off  period=1  equ=P=C  opselect=C  inp2=PCIN>>17  opr=+  inp1=P  carry=CIN  dbl_ovrd=off  block_type=constant
  Constant3 : xbsIndex_r4/Constant  const=0  gui_display_data_type=Floating-point  arith_type=Floating-point  n_bits=16  bin_pt=14  preci_type=Double  exp_width=8  frac_width=24  explicit_period=off  period=1  equ=P=C  opselect=C  inp2=PCIN>>17  opr=+  inp1=P  carry=CIN  dbl_ovrd=off  block_type=constant
  Constant4 : xbsIndex_r4/Constant  const=5  gui_display_data_type=Floating-point  arith_type=Floating-point  n_bits=16  bin_pt=14  preci_type=Double  exp_width=8  frac_width=24  explicit_period=off  period=1  equ=P=C  opselect=C  inp2=PCIN>>17  opr=+  inp1=P  carry=CIN  dbl_ovrd=off  block_type=constant
  Logical : xbsIndex_r4/Logical  logical_function=OR  inputs=2  en=off  latency=1  precision=Full  arith_type=Unsigned  n_bits=16  bin_pt=0  align_bp=on  dbl_ovrd=off  block_type=logical
  Mux : xbsIndex_r4/Mux  inputs=2  en=off  latency=1  precision=Full  arith_type=Unsigned  n_bits=16  bin_pt=14  quantization=Truncate  overflow=Wrap  dbl_ovrd=off  block_type=mux
  Mux1 : xbsIndex_r4/Mux  inputs=2  en=off  latency=1  precision=Full  arith_type=Unsigned  n_bits=16  bin_pt=14  quantization=Truncate  overflow=Wrap  dbl_ovrd=off  block_type=mux
  Relational : xbsIndex_r4/Relational  mode=a<b  op_type=Bool  en=off  latency=1  dbl_ovrd=off  block_type=relational
  Relational1 : xbsIndex_r4/Relational  mode=a>b  op_type=Bool  en=off  latency=1  dbl_ovrd=off  block_type=relational
  Relational2 : xbsIndex_r4/Relational  mode=a<b  op_type=Bool  en=off  latency=1  dbl_ovrd=off  block_type=relational
  PS : Outport
  wires:
  Constant1/1 -> Relational1/2
  Mux/1 -> PS/1
  Logical/1 -> Mux/1
  Relational/1 -> Logical/1
  Constant/1 -> Relational/2
  Constant3/1 -> Mux/3
  Relational1/1 -> Logical/2
  Constant2/1 -> AddSub/2
  AddSub/1 -> CMult/1
  Constant4/1 -> Relational2/2
  Relational2/1 -> Mux1/1
  e/1 -> Relational2/1, CMult1/1, AddSub/1, Relational1/1, Relational/1
  CMult1/1 -> Mux1/3
  CMult/1 -> Mux1/2
  Mux1/1 -> Mux/2

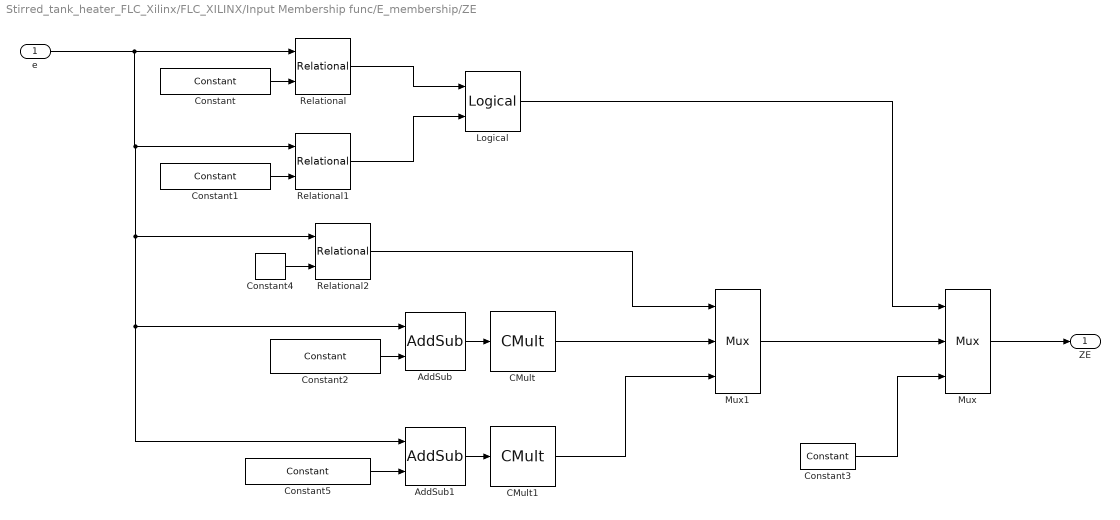
== system Stirred_tank_heater_FLC_Xilinx/FLC_XILINX/Input Membership func/E_membership/ZE ==
  e : Inport
  AddSub : xbsIndex_r4/AddSub  mode=Subtraction  use_carryin=off  use_carryout=off  en=off  latency=1  precision=Full  arith_type=Unsigned  n_bits=16  bin_pt=14  quantization=Truncate  overflow=Wrap  use_behavioral_HDL=off  hw_selection=Fabric  pipelined=off  dbl_ovrd=off  block_type=addsub
  AddSub1 : xbsIndex_r4/AddSub  mode=Addition  use_carryin=off  use_carryout=off  en=off  latency=1  precision=Full  arith_type=Unsigned  n_bits=16  bin_pt=14  quantization=Truncate  overflow=Wrap  use_behavioral_HDL=off  hw_selection=Fabric  pipelined=off  dbl_ovrd=off  block_type=addsub
  CMult : xbsIndex_r4/CMult  const=-1/5  gui_display_data_type=Floating-point  const_n_bits=16  const_bin_pt=14  float_type=Double  exp_bits=8  fraction_bits=24  en=off  latency=1  precision=Full  arith_type="Signed  (2's comp)"  n_bits=16  bin_pt=14  quantization=Truncate  overflow=Wrap  use_behavioral_HDL=off  mem_type=Distributed RAM  pipeline=off  dbl_ovrd=off  block_type=cmult
  CMult1 : xbsIndex_r4/CMult  const=1/5  gui_display_data_type=Floating-point  const_n_bits=16  const_bin_pt=14  float_type=Double  exp_bits=8  fraction_bits=24  en=off  latency=1  precision=Full  arith_type="Signed  (2's comp)"  n_bits=16  bin_pt=14  quantization=Truncate  overflow=Wrap  use_behavioral_HDL=off  mem_type=Distributed RAM  pipeline=off  dbl_ovrd=off  block_type=cmult
  Constant : xbsIndex_r4/Constant  const=-5  gui_display_data_type=Floating-point  arith_type=Floating-point  n_bits=16  bin_pt=14  preci_type=Double  exp_width=8  frac_width=24  explicit_period=off  period=1  equ=P=C  opselect=C  inp2=PCIN>>17  opr=+  inp1=P  carry=CIN  dbl_ovrd=off  block_type=constant
  Constant1 : xbsIndex_r4/Constant  const=5  gui_display_data_type=Floating-point  arith_type=Floating-point  n_bits=16  bin_pt=14  preci_type=Double  exp_width=8  frac_width=24  explicit_period=off  period=1  equ=P=C  opselect=C  inp2=PCIN>>17  opr=+  inp1=P  carry=CIN  dbl_ovrd=off  block_type=constant
  Constant2 : xbsIndex_r4/Constant  const=5  gui_display_data_type=Floating-point  arith_type=Floating-point  n_bits=16  bin_pt=14  preci_type=Double  exp_width=8  frac_width=24  explicit_period=off  period=1  equ=P=C  opselect=C  inp2=PCIN>>17  opr=+  inp1=P  carry=CIN  dbl_ovrd=off  block_type=constant
  Constant3 : xbsIndex_r4/Constant  const=0  gui_display_data_type=Floating-point  arith_type=Floating-point  n_bits=16  bin_pt=14  preci_type=Double  exp_width=8  frac_width=24  explicit_period=off  period=1  equ=P=C  opselect=C  inp2=PCIN>>17  opr=+  inp1=P  carry=CIN  dbl_ovrd=off  block_type=constant
  Constant4 : xbsIndex_r4/Constant  const=0  gui_display_data_type=Floating-point  arith_type=Floating-point  n_bits=16  bin_pt=14  preci_type=Double  exp_width=8  frac_width=24  explicit_period=off  period=1  equ=P=C  opselect=C  inp2=PCIN>>17  opr=+  inp1=P  carry=CIN  dbl_ovrd=off  block_type=constant
  Constant5 : xbsIndex_r4/Constant  const=5  gui_display_data_type=Floating-point  arith_type=Floating-point  n_bits=16  bin_pt=14  preci_type=Double  exp_width=8  frac_width=24  explicit_period=off  period=1  equ=P=C  opselect=C  inp2=PCIN>>17  opr=+  inp1=P  carry=CIN  dbl_ovrd=off  block_type=constant
  Logical : xbsIndex_r4/Logical  logical_function=OR  inputs=2  en=off  latency=1  precision=Full  arith_type=Unsigned  n_bits=16  bin_pt=0  align_bp=on  dbl_ovrd=off  block_type=logical
  Mux : xbsIndex_r4/Mux  inputs=2  en=off  latency=1  precision=Full  arith_type=Unsigned  n_bits=16  bin_pt=14  quantization=Truncate  overflow=Wrap  dbl_ovrd=off  block_type=mux
  Mux1 : xbsIndex_r4/Mux  inputs=2  en=off  latency=1  precision=Full  arith_type=Unsigned  n_bits=16  bin_pt=14  quantization=Truncate  overflow=Wrap  dbl_ovrd=off  block_type=mux
  Relational : xbsIndex_r4/Relational  mode=a<b  op_type=Bool  en=off  latency=1  dbl_ovrd=off  block_type=relational
  Relational1 : xbsIndex_r4/Relational  mode=a>b  op_type=Bool  en=off  latency=1  dbl_ovrd=off  block_type=relational
  Relational2 : xbsIndex_r4/Relational  mode=a<b  op_type=Bool  en=off  latency=1  dbl_ovrd=off  block_type=relational
  ZE : Outport
  wires:
  Constant1/1 -> Relational1/2
  Mux/1 -> ZE/1
  Logical/1 -> Mux/1
  Relational/1 -> Logical/1
  Constant/1 -> Relational/2
  Constant3/1 -> Mux/3
  Relational1/1 -> Logical/2
  Constant2/1 -> AddSub/2
  AddSub/1 -> CMult/1
  Constant4/1 -> Relational2/2
  Relational2/1 -> Mux1/1
  AddSub1/1 -> CMult1/1
  Constant5/1 -> AddSub1/2
  e/1 -> Relational2/1, AddSub1/1, AddSub/1, Relational1/1, Relational/1
  CMult1/1 -> Mux1/3
  CMult/1 -> Mux1/2
  Mux1/1 -> Mux/2

== system Stirred_tank_heater_FLC_Xilinx/FLC_XILINX/Input Membership func/IE_membership/NB ==
  de : Inport
  AddSub : xbsIndex_r4/AddSub  mode=Addition  use_carryin=off  use_carryout=off  en=off  latency=1  precision=Full  arith_type=Unsigned  n_bits=16  bin_pt=14  quantization=Truncate  overflow=Wrap  use_behavioral_HDL=off  hw_selection=Fabric  pipelined=off  dbl_ovrd=off  block_type=addsub
  CMult : xbsIndex_r4/CMult  const=-1/5  gui_display_data_type=Floating-point  const_n_bits=16  const_bin_pt=14  float_type=Double  exp_bits=8  fraction_bits=24  en=off  latency=1  precision=Full  arith_type="Signed  (2's comp)"  n_bits=16  bin_pt=14  quantization=Truncate  overflow=Wrap  use_behavioral_HDL=off  mem_type=Distributed RAM  pipeline=off  dbl_ovrd=off  block_type=cmult
  Constant : xbsIndex_r4/Constant  const=-10  gui_display_data_type=Floating-point  arith_type=Floating-point  n_bits=16  bin_pt=14  preci_type=Double  exp_width=8  frac_width=24  explicit_period=off  period=1  equ=P=C  opselect=C  inp2=PCIN>>17  opr=+  inp1=P  carry=CIN  dbl_ovrd=off  block_type=constant
  Constant1 : xbsIndex_r4/Constant  const=-5  gui_display_data_type=Floating-point  arith_type=Floating-point  n_bits=16  bin_pt=14  preci_type=Double  exp_width=8  frac_width=24  explicit_period=off  period=1  equ=P=C  opselect=C  inp2=PCIN>>17  opr=+  inp1=P  carry=CIN  dbl_ovrd=off  block_type=constant
  Constant2 : xbsIndex_r4/Constant  const=5  gui_display_data_type=Floating-point  arith_type=Floating-point  n_bits=16  bin_pt=14  preci_type=Double  exp_width=8  frac_width=24  explicit_period=off  period=1  equ=P=C  opselect=C  inp2=PCIN>>17  opr=+  inp1=P  carry=CIN  dbl_ovrd=off  block_type=constant
  Constant3 : xbsIndex_r4/Constant  const=0  gui_display_data_type=Floating-point  arith_type=Floating-point  n_bits=16  bin_pt=14  preci_type=Double  exp_width=8  frac_width=24  explicit_period=off  period=1  equ=P=C  opselect=C  inp2=PCIN>>17  opr=+  inp1=P  carry=CIN  dbl_ovrd=off  block_type=constant
  Logical : xbsIndex_r4/Logical  logical_function=OR  inputs=2  en=off  latency=1  precision=Full  arith_type=Unsigned  n_bits=16  bin_pt=0  align_bp=on  dbl_ovrd=off  block_type=logical
  Mux : xbsIndex_r4/Mux  inputs=2  en=off  latency=1  precision=Full  arith_type=Unsigned  n_bits=16  bin_pt=14  quantization=Truncate  overflow=Wrap  dbl_ovrd=off  block_type=mux
  Relational : xbsIndex_r4/Relational  mode=a<b  op_type=Bool  en=off  latency=1  dbl_ovrd=off  block_type=relational
  Relational1 : xbsIndex_r4/Relational  mode=a>b  op_type=Bool  en=off  latency=1  dbl_ovrd=off  block_type=relational
  NB : Outport
  wires:
  CMult/1 -> Mux/2
  de/1 -> AddSub/1, Relational1/1, Relational/1
  Constant1/1 -> Relational1/2
  Mux/1 -> NB/1
  Logical/1 -> Mux/1
  Relational/1 -> Logical/1
  Constant/1 -> Relational/2
  Constant3/1 -> Mux/3
  Relational1/1 -> Logical/2
  Constant2/1 -> AddSub/2
  AddSub/1 -> CMult/1
